simulink subsystem "Engine"  (R2025a)
settings: Solver=VariableStepAuto  StartTime=0.0  StopTime=10.0  RelTol=1e-3
libraries: fl_lib x12, nesl_utility x11
settings Model: Creator=Adam  LastModifiedBy=mu22504

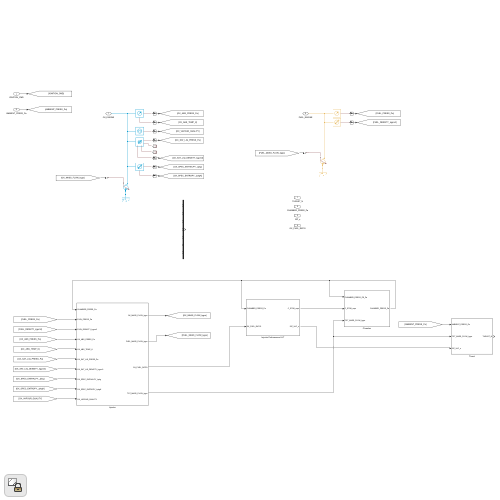
[thumbnail: Simulink's stored preview of the top-level diagram]
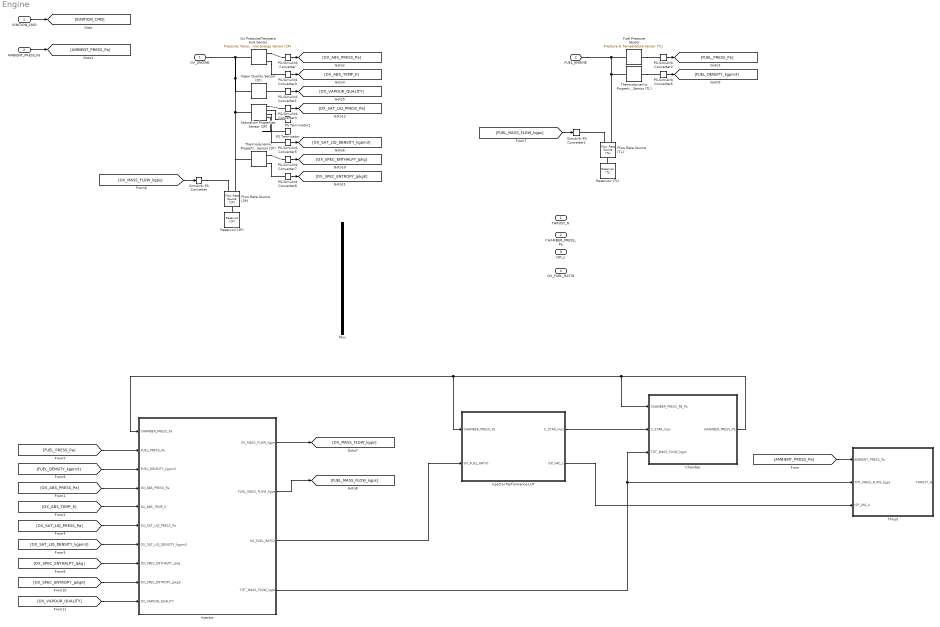
== system Engine ==
  "IGNITION_CMD " : Inport
  AMBIENT_PRESS_Pa : Inport  Port=2
  Chamber : Subsystem
  Flow Rate Source (2P) : fl_lib/Two-Phase Fluid/Sources/Flow Rate Source (2P)  source_type=foundation.enum.constant_controlled.controlled  flow_type=foundation.enum.mass_volumetric_flow.mass  mass_flow=0 kg/s  volumetric_flow=0 m^3/s  power_spec=foundation.enum.power_spec.isentropic  area_A=0.01 m^2  area_B=0.01 m^2
      settings: InternalSimscapePortConfiguration="{\"Bottom\":[],\"Left\":[{\"id\":\"A\",\"label\":\"A\",\"type\":\"foundation.two_phase_fluid.two_phase_fluid\"},{\"id\":\"M\",\"label\":\"M\",\"type\":\"input\"}],\"Right\":[{\"id\":\"B\",\"label\":\"B\",\"type\":\"foundation.two_phase_fluid.two_phase_fluid\"}],\"Top\":[]}"
  Flow Rate Source (TL) : fl_lib/Thermal Liquid/Sources/Flow Rate Source (TL)  source_type=foundation.enum.constant_controlled.controlled  flow_type=foundation.enum.mass_volumetric_flow.mass  mass_flow=0 kg/s  volumetric_flow=0 m^3/s  power_spec=foundation.enum.power_spec.isentropic  area=0.01 m^2
  Fuel Pressure Sensor : fl_lib/Thermal Liquid/Sensors/Pressure & Temperature Sensor (TL)  reference=foundation.enum.MeasurementReference.absolute  pressure=true  pressure_spec=foundation.enum.PressureMeasementSpec.Absolute  temperature=false
      settings: InternalSimscapePortConfiguration="{\"Bottom\":[],\"Left\":[{\"id\":\"A\",\"label\":\"A\",\"type\":\"foundation.thermal_liquid.thermal_liquid\"}],\"Right\":[{\"id\":\"Pa\",\"label\":\"Pa\",\"type\":\"output\"}],\"Top\":[]}"
  Injector : Subsystem
  Injector Performance LUT : Subsystem
  Mux : Mux  Inputs=7
  Ox Pressure/Temperature Sensor : fl_lib/Two-Phase Fluid/Sensors/Pressure, Temperature & Internal Energy Sensor (2P)  reference=foundation.enum.MeasurementReference.absolute  pressure=true  pressure_spec=foundation.enum.PressureMeasementSpec.Absolute  temperature=true  internal_energy=false
      settings: InternalSimscapePortConfiguration="{\"Bottom\":[{\"id\":\"T\",\"label\":\"T\",\"type\":\"output\"}],\"Left\":[{\"id\":\"A\",\"label\":\"A\",\"type\":\"foundation.two_phase_fluid.two_phase_fluid\"}],\"Right\":[{\"id\":\"Pa\",\"label\":\"Pa\",\"type\":\"output\"}],\"Top\":[]}"
  PS Terminator : fl_lib/Physical Signals/Sinks/PS Terminator
  PS Terminator1 : fl_lib/Physical Signals/Sinks/PS Terminator
  PS-Simulink Converter : nesl_utility/PS-Simulink Converter  PhysicalDomain=network_engine_domain  SubClassName=ps_output  LeftPortType=input  RightPortType=output  PseudoPeriodic=off  Frequencies=[]  VectorFormat=inherit  Unit=Pa  AffineConversion=off
  PS-Simulink Converter1 : nesl_utility/PS-Simulink Converter  PhysicalDomain=network_engine_domain  SubClassName=ps_output  LeftPortType=input  RightPortType=output  PseudoPeriodic=off  Frequencies=[]  VectorFormat=inherit  Unit=inherit  AffineConversion=off
  PS-Simulink Converter2 : nesl_utility/PS-Simulink Converter  PhysicalDomain=network_engine_domain  SubClassName=ps_output  LeftPortType=input  RightPortType=output  PseudoPeriodic=off  Frequencies=[]  VectorFormat=inherit  Unit=Pa  AffineConversion=off
  PS-Simulink Converter3 : nesl_utility/PS-Simulink Converter  PhysicalDomain=network_engine_domain  SubClassName=ps_output  LeftPortType=input  RightPortType=output  PseudoPeriodic=off  Frequencies=[]  VectorFormat=inherit  Unit=K  AffineConversion=off
  PS-Simulink Converter4 : nesl_utility/PS-Simulink Converter  PhysicalDomain=network_engine_domain  SubClassName=ps_output  LeftPortType=input  RightPortType=output  PseudoPeriodic=off  Frequencies=[]  VectorFormat=inherit  Unit=Pa  AffineConversion=off
  PS-Simulink Converter5 : nesl_utility/PS-Simulink Converter  PhysicalDomain=network_engine_domain  SubClassName=ps_output  LeftPortType=input  RightPortType=output  PseudoPeriodic=off  Frequencies=[]  VectorFormat=inherit  Unit=kg/m^3  AffineConversion=off
  PS-Simulink Converter6 : nesl_utility/PS-Simulink Converter  PhysicalDomain=network_engine_domain  SubClassName=ps_output  LeftPortType=input  RightPortType=output  PseudoPeriodic=off  Frequencies=[]  VectorFormat=inherit  Unit=kg/m^3  AffineConversion=off
  PS-Simulink Converter7 : nesl_utility/PS-Simulink Converter  PhysicalDomain=network_engine_domain  SubClassName=ps_output  LeftPortType=input  RightPortType=output  PseudoPeriodic=off  Frequencies=[]  VectorFormat=inherit  Unit=J/(kg*K)  AffineConversion=off
  PS-Simulink Converter8 : nesl_utility/PS-Simulink Converter  PhysicalDomain=network_engine_domain  SubClassName=ps_output  LeftPortType=input  RightPortType=output  PseudoPeriodic=off  Frequencies=[]  VectorFormat=inherit  Unit=J/(kg*K)  AffineConversion=off
  Reservoir (2P) : fl_lib/Two-Phase Fluid/Elements/Reservoir (2P)  pressure_spec=foundation.enum.ReservoirPressureSpec2P.Atmospheric  reservoir_pressure=0.101325 MPa  reservoir_condensing_temperature=373.15 K  reservoir_evaporating_temperature=373.15 K  energy_spec=foundation.enum.ReservoirEnergySpec2P.Temperature  reservoir_temperature=293.15 K  reservoir_quality=0.5  reservoir_void_fraction=0.5  reservoir_enthalpy=1500 kJ/kg  reservoir_internal_energy=1500 kJ/kg  reservoir_subcooling=5 deltaK  reservoir_superheating=5 deltaK  area_A=0.01 m^2
  Reservoir (TL) : fl_lib/Thermal Liquid/Elements/Reservoir (TL)  pressure_spec=foundation.enum.pressure_spec.atmospheric  reservoir_pressure=0.101325 MPa  reservoir_temperature=293.15 K  area=0.01 m^2
  Saturation Properties Sensor (2P) : fl_lib/Two-Phase Fluid/Sensors/Saturation Properties Sensor (2P)  temperature_measure=false  pressure_measure=true  pressure_check=simscape.enum.assert.action.warn  energy_measure=foundation.enum.EnergyMeasurement.Off  density_measure=foundation.enum.DensityMeasurement.SaturatedDensity
      settings: InternalSimscapePortConfiguration="{\"Bottom\":[{\"id\":\"rho_sat_liq\",\"label\":\"rhoL\",\"type\":\"output\"},{\"id\":\"rho_sat_vap\",\"label\":\"rhoV\",\"type\":\"output\"}],\"Left\":[{\"id\":\"A\",\"label\":\"A\",\"type\":\"foundation.two_phase_fluid.two_phase_fluid\"}],\"Right\":[{\"id\":\"p_sat_liq\",\"label\":\"PL\",\"type\":\"output\"},{\"id\":\"p_sat_vap\",\"label\":\"PV\",\"type\":\"output\"}],\"Top\":[]}"
  Simulink-PS Converter : nesl_utility/Simulink-PS Converter  PhysicalDomain=network_engine_domain  SubClassName=ps_input  LeftPortType=input  RightPortType=output  PseudoPeriodic=off  Frequencies=[]  NoiseDistribution=none  NoiseParameters=[]  Unit=kg/s  AffineConversion=off  FilteringAndDerivatives=provide  SimscapeFilterOrder=1  InputFilterTimeConstant=0.001  UdotUserProvided=0
  Simulink-PS Converter1 : nesl_utility/Simulink-PS Converter  PhysicalDomain=network_engine_domain  SubClassName=ps_input  LeftPortType=input  RightPortType=output  PseudoPeriodic=off  Frequencies=[]  NoiseDistribution=none  NoiseParameters=[]  Unit=kg/s  AffineConversion=off  FilteringAndDerivatives=provide  SimscapeFilterOrder=1  InputFilterTimeConstant=0.001  UdotUserProvided=0
  Thermodynamic Properties Sensor (2P) : fl_lib/Two-Phase Fluid/Sensors/Thermodynamic Properties Sensor (2P)  temperature=false  enthalpy=true  density=false  specific_volume=false  entropy=true
      settings: InternalSimscapePortConfiguration="{\"Bottom\":[{\"id\":\"S\",\"label\":\"s\",\"type\":\"output\"}],\"Left\":[{\"id\":\"A\",\"label\":\"A\",\"type\":\"foundation.two_phase_fluid.two_phase_fluid\"}],\"Right\":[{\"id\":\"H\",\"label\":\"h\",\"type\":\"output\"}],\"Top\":[]}"
  Thermodynamic Properties Sensor (TL) : fl_lib/Thermal Liquid/Sensors/Thermodynamic Properties Sensor (TL)  internal_energy=false  density=true  specific_heat=false
      settings: InternalSimscapePortConfiguration="{\"Bottom\":[],\"Left\":[{\"id\":\"A\",\"label\":\"A\",\"type\":\"foundation.thermal_liquid.thermal_liquid\"}],\"Right\":[{\"id\":\"RHO\",\"label\":\"ρ\",\"type\":\"output\"}],\"Top\":[]}"
  Thrust : Subsystem
  Vapor Quality Sensor (2P) : fl_lib/Two-Phase Fluid/Sensors/Vapor Quality Sensor (2P)  vapor_fraction_spec=foundation.enum.vapor_fraction_spec.quality
      settings: InternalSimscapePortConfiguration="{\"Bottom\":[],\"Left\":[{\"id\":\"A\",\"label\":\"A\",\"type\":\"foundation.two_phase_fluid.two_phase_fluid\"}],\"Right\":[{\"id\":\"X\",\"label\":\"X\",\"type\":\"output\"}],\"Top\":[]}"
  OX_ENGINE : PMIOPort  Side=Left
  FUEL_ENGINE : PMIOPort  Port=2  Side=Left
  THRUST_N : Outport
  CHAMBER_PRESS_Pa : Outport  Port=2
  ISP_s : Outport  Port=3
  OX_FUEL_RATIO : Outport  Port=4
  wires:
  Injector/3(OX_FUEL_RATIO) -> Injector Performance LUT/2(OX_FUEL_RATIO)
  Injector Performance LUT/1(C_STAR_mps) -> Chamber/2(C_STAR_mps)
  Injector Performance LUT/2(ISP_VAC_s) -> Thrust/3(ISP_VAC_s)
  Injector/4(TOT_MASS_FLOW_kgps) -> Thrust/2(TOT_MASS_FLOW_kgps), Chamber/3(TOT_MASS_FLOW_kgps)
  AMBIENT_PRESS_Pa/1 -> [AMBIENT_PRESS_Pa]
  "IGNITION_CMD "/1 -> [IGNITION_CMD]
  [AMBIENT_PRESS_Pa] -> Thrust/1(AMBIENT_PRESS_Pa)
  Chamber/1(CHAMBER_PRESS_Pa) -> Injector/1(CHAMBER_PRESS_Pa), Injector Performance LUT/1(CHAMBER_PRESS_Pa), Chamber/1(CHAMBER_PRESS_FB_Pa)
  PS-Simulink Converter/1 -> [OX_ABS_PRESS_Pa]
  PS-Simulink Converter1/1 -> [OX_VAPOUR_QUALITY]
  PS-Simulink Converter2/1 -> [FUEL_PRESS_Pa]
  PS-Simulink Converter3/1 -> [OX_ABS_TEMP_K]
  PS-Simulink Converter5/1 -> [OX_SAT_LIQ_DENSITY_kgpm3]
  [FUEL_PRESS_Pa] -> Injector/2(FUEL_PRESS_Pa)
  Injector/1(OX_MASS_FLOW_kgps) -> [OX_MASS_FLOW_kgps]
  Injector/2(FUEL_MASS_FLOW_kgps) -> [FUEL_MASS_FLOW_kgps]
  [OX_MASS_FLOW_kgps] -> Simulink-PS Converter/1
  [FUEL_MASS_FLOW_kgps] -> Simulink-PS Converter1/1
  PS-Simulink Converter6/1 -> [FUEL_DENSITY_kgpm3]
  PS-Simulink Converter7/1 -> [OX_SPEC_ENTHALPY_Jpkg]
  PS-Simulink Converter8/1 -> [OX_SPEC_ENTROPY_JpkgK]
  PS-Simulink Converter4/1 -> [OX_SAT_LIQ_PRESS_Pa]
  [FUEL_DENSITY_kgpm3] -> Injector/3(FUEL_DENSITY_kgpm3)
  [OX_ABS_PRESS_Pa] -> Injector/4(OX_ABS_PRESS_Pa)
  [OX_ABS_TEMP_K] -> Injector/5(OX_ABS_TEMP_K)
  [OX_SAT_LIQ_PRESS_Pa] -> Injector/6(OX_SAT_LIQ_PRESS_Pa)
  [OX_SAT_LIQ_DENSITY_kgpm3] -> Injector/7(OX_SAT_LIQ_DENSITY_kgpm3)
  [OX_SPEC_ENTHALPY_Jpkg] -> Injector/8(OX_SPEC_ENTHALPY_Jpkg)
  [OX_SPEC_ENTROPY_JpkgK] -> Injector/9(OX_SPEC_ENTROPY_JpkgK)
  [OX_VAPOUR_QUALITY] -> Injector/10(OX_VAPOUR_QUALITY)
  connections:
  FUEL_ENGINE/RConn1 -- Flow Rate Source (TL)/LConn1 -- Thermodynamic Properties Sensor (TL)/LConn1 -- Fuel Pressure Sensor/LConn1
  OX_ENGINE/RConn1 -- Ox Pressure/Temperature Sensor/LConn1 -- Saturation Properties Sensor (2P)/LConn1 -- Thermodynamic Properties Sensor (2P)/LConn1 -- Flow Rate Source (2P)/LConn1 -- Vapor Quality Sensor (2P)/LConn1
  Ox Pressure/Temperature Sensor/RConn1 -- PS-Simulink Converter/LConn1
  PS-Simulink Converter1/LConn1 -- Vapor Quality Sensor (2P)/RConn1
  Fuel Pressure Sensor/RConn1 -- PS-Simulink Converter2/LConn1
  Ox Pressure/Temperature Sensor/RConn2 -- PS-Simulink Converter3/LConn1
  PS Terminator/LConn1 -- Saturation Properties Sensor (2P)/RConn4
  Saturation Properties Sensor (2P)/RConn3 -- PS-Simulink Converter5/LConn1
  Flow Rate Source (TL)/RConn1 -- Reservoir (TL)/LConn1
  Flow Rate Source (2P)/RConn1 -- Reservoir (2P)/LConn1
  Simulink-PS Converter/RConn1 -- Flow Rate Source (2P)/LConn2
  Simulink-PS Converter1/RConn1 -- Flow Rate Source (TL)/LConn2
  Thermodynamic Properties Sensor (TL)/RConn1 -- PS-Simulink Converter6/LConn1
  Thermodynamic Properties Sensor (2P)/RConn1 -- PS-Simulink Converter7/LConn1
  Thermodynamic Properties Sensor (2P)/RConn2 -- PS-Simulink Converter8/LConn1
  Saturation Properties Sensor (2P)/RConn2 -- PS Terminator1/LConn1
  PS-Simulink Converter4/LConn1 -- Saturation Properties Sensor (2P)/RConn1

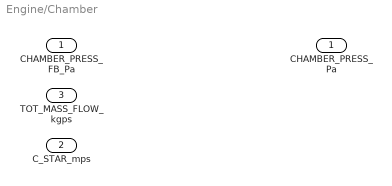
== system Engine/Chamber ==
  CHAMBER_PRESS_FB_Pa : Inport
  C_STAR_mps : Inport  Port=2
  TOT_MASS_FLOW_kgps : Inport  Port=3
  CHAMBER_PRESS_Pa : Outport

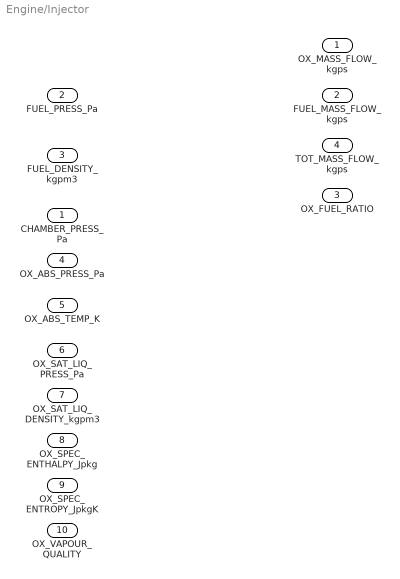
== system Engine/Injector ==
  CHAMBER_PRESS_Pa : Inport
  FUEL_PRESS_Pa : Inport  Port=2
  FUEL_DENSITY_kgpm3 : Inport  Port=3
  OX_ABS_PRESS_Pa : Inport  Port=4
  OX_ABS_TEMP_K : Inport  Port=5
  OX_SAT_LIQ_PRESS_Pa : Inport  Port=6
  OX_SAT_LIQ_DENSITY_kgpm3 : Inport  Port=7
  OX_SPEC_ENTHALPY_Jpkg : Inport  Port=8
  OX_SPEC_ENTROPY_JpkgK : Inport  Port=9
  OX_VAPOUR_QUALITY : Inport  Port=10
  OX_MASS_FLOW_kgps : Outport
  FUEL_MASS_FLOW_kgps : Outport  Port=2
  OX_FUEL_RATIO : Outport  Port=3
  TOT_MASS_FLOW_kgps : Outport  Port=4

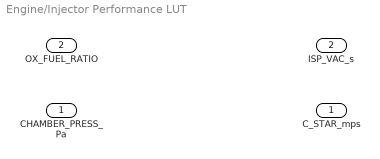
== system Engine/Injector Performance LUT ==
  CHAMBER_PRESS_Pa : Inport
  OX_FUEL_RATIO : Inport  Port=2
  C_STAR_mps : Outport
  ISP_VAC_s : Outport  Port=2

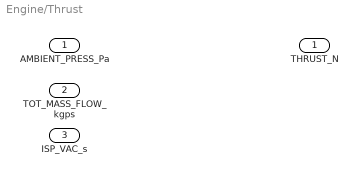
== system Engine/Thrust ==
  AMBIENT_PRESS_Pa : Inport
  TOT_MASS_FLOW_kgps : Inport  Port=2
  ISP_VAC_s : Inport  Port=3
  THRUST_N : Outport
